simulink model "TrialAOOR"  (R2021a)
settings: Solver=FixedStepAuto  StartTime=0.0  StopTime=50  FixedStep=1e-3  RelTol=1e-3  EnableMultiTasking=on
undefined symbols (not defined in the file): D0, D1, D10, D11, D12, D13, D2, D3, D4, D5, D6, D7, D8, D9, magnitude, PTA0, PTA1, PTA2, PTB23, PTB9, PTC16, PTC17, PTC2, PTC3, PTC4, PTD0, PTD1, PTD2, PTD3
libraries: frdmk64flib x19, dspstat3 x1
settings Model: PacingRate=0.250000  ExtModeTrigDuration=5  Creator=Arun Mistry  LastModifiedBy=Arun Mistry
settings OptimizationCC: EnhancedBackFolding=on  PassReuseOutputArgsAs=Individual arguments  ZeroExternalMemoryAtStartup=off  ZeroInternalMemoryAtStartup=off  MaxStackSize=64  OptimizeBlockOrder=speed  DifferentSizesBufferReuse=on  OptimizationCustomize=off  EfficientTunableParamExpr=on
settings DebuggingCC: ParameterTunabilityLossMsg=error
settings HardwareCC: ProdBitPerPointer=32  ProdBitPerSizeT=32  ProdBitPerPtrDiffT=32  ProdLargestAtomicInteger=Long  ProdLargestAtomicFloat=Double  ProdWordSize=32  ProdHWDeviceType=ARM Compatible->ARM Cortex
settings SFSimCC: MATLABDynamicMemAlloc=off
settings RTWCC: SystemTargetFile=ert.tlc  HardwareBoard=NXP FRDM-K64F  TLCOptions="-aInlineSetEventsForThisBaseRateFcn=TLC_FALSE -aSuppressMultiTaskScheduler=TLC_FALSE  -aRateBasedStepFcn=0"  TemplateMakefile=ert_default_tmf  Toolchain=GNU Tools for ARM Embedded Processors
settings CodeAppCC: ForceParamTrailComments=on  IgnoreCustomStorageClasses=off  OperatorAnnotations=on  SimulinkDataObjDesc=on  SFDataObjDesc=on  InsertBlockDesc=on
settings ERTTargetCC: ExtModeTransport=4  ExtModeMexFile=sendToCommService

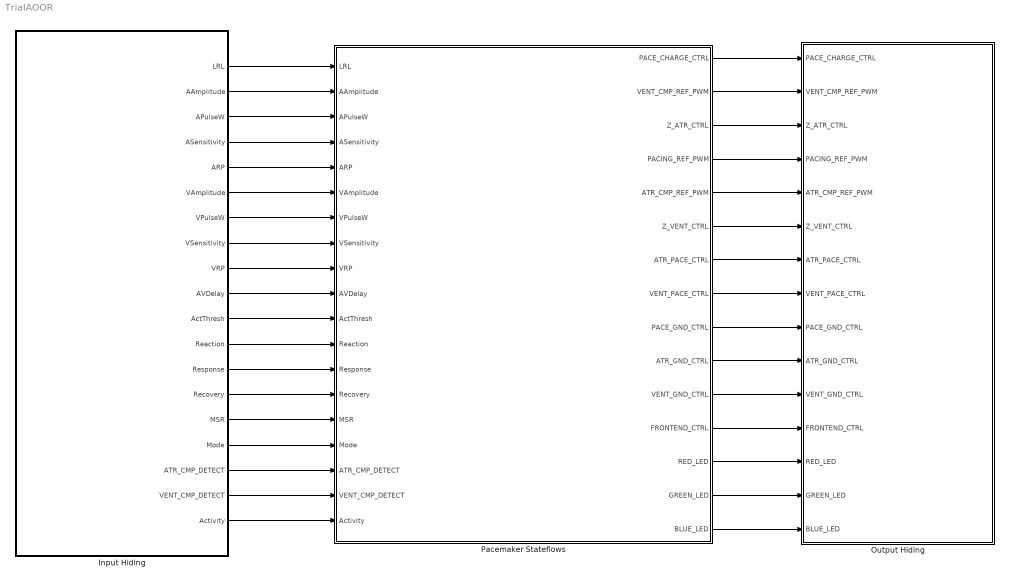
== system TrialAOOR ==
  Input Hiding : Subsystem
  Output Hiding : Subsystem
  Pacemaker Stateflows : Stateflow chart  TreatAsAtomicUnit=on
      settings: PortSchema="{\"entries\":[{\"content\":{\"sides\":[{\"content\":{\"connectorIds\":[\"In1\",\"In2\",\"In3\",\"In4\",\"In5\",\"In6\",\"In7\",\"In8\",\"In9\",\"In17\",\"In11\",\"In10\",\"In12\",\"In14\",\"In19\",\"In13\",\"In15\",\"In16\",\"In18\"]},\"type\":\"ConnectorPlacement.EquallySpacedRectSide\",\"uuid\":\"6f24296b-9994-4871-8227-e053a3629335\"},{\"content\":{\"connectorIds\":[\"Out1\",\"Out2\",\"Out3\",\"Out4\",\"Out5\",\"Out6\",\"Out7\",\"Out8\",\"Out9\",\"Out10\",\"Out11\",\"Out12\",\"Out13\",\"Out14\",\"Out15\"],\"side\":\"RIGHT\"},\"type\":\"ConnectorPlacement.EquallySpacedRectSide\",\"uuid\":\"36cf1f29-c3ea-48aa-b003-da737efff16a\"},{\"content\":{\"connectorIds\":[],\"side\":\"TOP\"},\"type\":\"ConnectorPlacement.EquallySpacedRectSide\",\"uuid\":\"8330eb51-0bc3-4d96-96ed-331fbb159cdb\"}]},\"type\":\"ConnectorPlacement.EquallySpacedConnector\",\"uuid\":\"1e79ed8a-065e-4a3c-97dd-23eb49490e0b\"}],\"packageUris\":[\"http://schema.mathworks.com/mf0/Connector/R2020b\"],\"version\":\"1.0\"}"
  wires:
  Pacemaker Stateflows/1(PACE_CHARGE_CTRL) -> Output Hiding/1(PACE_CHARGE_CTRL)
  Input Hiding/17(ATR_CMP_DETECT) -> Pacemaker Stateflows/15(ATR_CMP_DETECT)
  Input Hiding/7(VPulseW) -> Pacemaker Stateflows/7(VPulseW)
  Input Hiding/18(VENT_CMP_DETECT) -> Pacemaker Stateflows/16(VENT_CMP_DETECT)
  Pacemaker Stateflows/3(Z_ATR_CTRL) -> Output Hiding/3(Z_ATR_CTRL)
  Input Hiding/3(APulseW) -> Pacemaker Stateflows/3(APulseW)
  Pacemaker Stateflows/7(ATR_PACE_CTRL) -> Output Hiding/7(ATR_PACE_CTRL)
  Pacemaker Stateflows/10(ATR_GND_CTRL) -> Output Hiding/10(ATR_GND_CTRL)
  Input Hiding/16(Mode) -> Pacemaker Stateflows/13(Mode)
  Input Hiding/2(AAmplitude) -> Pacemaker Stateflows/2(AAmplitude)
  Input Hiding/6(VAmplitude) -> Pacemaker Stateflows/6(VAmplitude)
  Pacemaker Stateflows/6(Z_VENT_CTRL) -> Output Hiding/6(Z_VENT_CTRL)
  Pacemaker Stateflows/4(PACING_REF_PWM) -> Output Hiding/4(PACING_REF_PWM)
  Pacemaker Stateflows/11(VENT_GND_CTRL) -> Output Hiding/11(VENT_GND_CTRL)
  Pacemaker Stateflows/9(PACE_GND_CTRL) -> Output Hiding/9(PACE_GND_CTRL)
  Pacemaker Stateflows/8(VENT_PACE_CTRL) -> Output Hiding/8(VENT_PACE_CTRL)
  Input Hiding/1(LRL) -> Pacemaker Stateflows/1(LRL)
  Pacemaker Stateflows/15(BLUE_LED) -> Output Hiding/15(BLUE_LED)
  Input Hiding/4(ASensitivity) -> Pacemaker Stateflows/4(ASensitivity)
  Pacemaker Stateflows/12(FRONTEND_CTRL) -> Output Hiding/12(FRONTEND_CTRL)
  Input Hiding/9(VRP) -> Pacemaker Stateflows/9(VRP)
  Input Hiding/8(VSensitivity) -> Pacemaker Stateflows/8(VSensitivity)
  Input Hiding/5(ARP) -> Pacemaker Stateflows/5(ARP)
  Pacemaker Stateflows/14(GREEN_LED) -> Output Hiding/14(GREEN_LED)
  Pacemaker Stateflows/13(RED_LED) -> Output Hiding/13(RED_LED)
  Pacemaker Stateflows/5(ATR_CMP_REF_PWM) -> Output Hiding/5(ATR_CMP_REF_PWM)
  Pacemaker Stateflows/2(VENT_CMP_REF_PWM) -> Output Hiding/2(VENT_CMP_REF_PWM)
  Input Hiding/10(AVDelay) -> Pacemaker Stateflows/17(AVDelay)
  Input Hiding/19(Activity) -> Pacemaker Stateflows/18(Activity)
  Input Hiding/12(Reaction) -> Pacemaker Stateflows/10(Reaction)
  Input Hiding/13(Response) -> Pacemaker Stateflows/12(Response)
  Input Hiding/14(Recovery) -> Pacemaker Stateflows/14(Recovery)
  Input Hiding/15(MSR) -> Pacemaker Stateflows/19(MSR)
  Input Hiding/11(ActThresh) -> Pacemaker Stateflows/11(ActThresh)

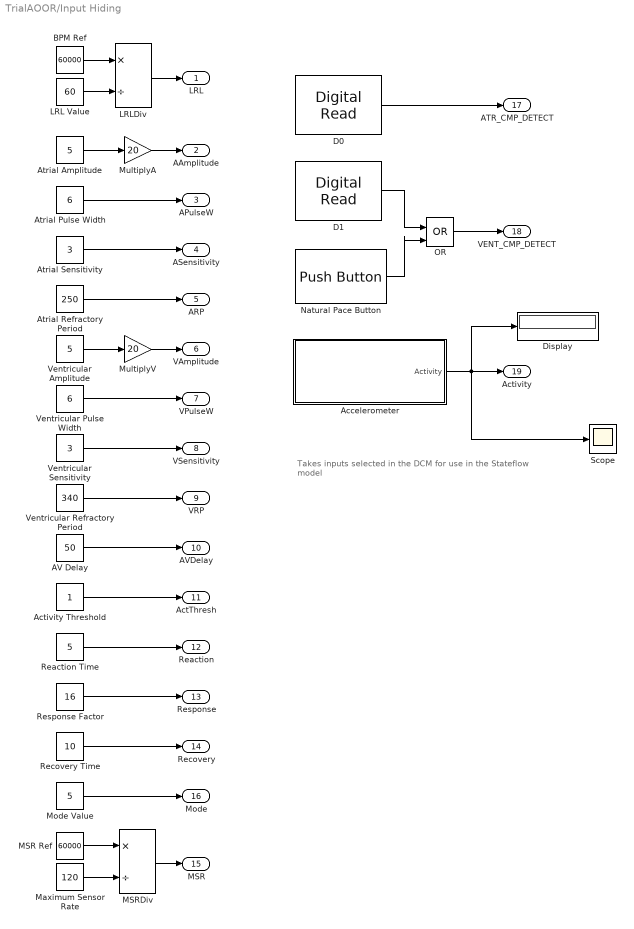
== system TrialAOOR/Input Hiding ==
  note: Takes inputs selected in the DCM for use in the Stateflow model
  AV Delay : Constant  Value=50  OutDataTypeStr=uint16
  Accelerometer : Subsystem
  Activity Threshold : Constant  OutDataTypeStr=double
  Atrial Amplitude : Constant  Value=5  OutDataTypeStr=uint16
  Atrial Pulse Width : Constant  Value=6  OutDataTypeStr=uint16
  Atrial Refractory Period : Constant  Value=250  OutDataTypeStr=uint16
  Atrial Sensitivity : Constant  Value=3  OutDataTypeStr=uint16
  BPM Ref : Constant  Value=60000  OutDataTypeStr=uint16
  D0 : frdmk64flib/Digital Read  Whichpin=PTC16 (D0)  SampleTime=-1
  D1 : frdmk64flib/Digital Read  Whichpin=PTC17 (D1)  SampleTime=-1
  Display : Display
  LRL Value : Constant  Value=60  OutDataTypeStr=uint16
  LRLDiv : Product  Inputs=*/  OutDataTypeStr=uint16  RndMeth=Round
  MSR Ref : Constant  Value=60000  OutDataTypeStr=uint16
  MSRDiv : Product  Inputs=*/  OutDataTypeStr=uint16  RndMeth=Round
  Maximum Sensor Rate : Constant  Value=120  OutDataTypeStr=uint16
  Mode Value : Constant  Value=5  OutDataTypeStr=uint16
  MultiplyA : Gain  Gain=20  OutDataTypeStr=uint16
  MultiplyV : Gain  Gain=20  OutDataTypeStr=uint16
  Natural Pace Button : frdmk64flib/Push Button  Whichswitch=SW3  SampleTime1=-1
  OR : Logic  Operator=OR  IconShape=distinctive  AllPortsSameDT=off  OutDataTypeStr=boolean
  Reaction Time : Constant  Value=5  OutDataTypeStr=uint16
  Recovery Time : Constant  Value=10  OutDataTypeStr=uint16
  Response Factor : Constant  Value=16  OutDataTypeStr=uint16
  Scope : Scope
  Ventricular Amplitude : Constant  Value=5  OutDataTypeStr=uint16
  Ventricular Pulse Width : Constant  Value=6  OutDataTypeStr=uint16
  Ventricular Refractory Period : Constant  Value=340  OutDataTypeStr=uint16
  Ventricular Sensitivity : Constant  Value=3  OutDataTypeStr=uint16
  LRL : Outport  OutDataTypeStr=uint16
  AAmplitude : Outport  Port=2  OutDataTypeStr=uint16
  APulseW : Outport  Port=3  OutDataTypeStr=uint16
  ASensitivity : Outport  Port=4  OutDataTypeStr=uint16
  ARP : Outport  Port=5  OutDataTypeStr=uint16
  VAmplitude : Outport  Port=6  OutDataTypeStr=uint16
  VPulseW : Outport  Port=7  OutDataTypeStr=uint16
  VSensitivity : Outport  Port=8  OutDataTypeStr=uint16
  VRP : Outport  Port=9  OutDataTypeStr=uint16
  AVDelay : Outport  Port=10  OutDataTypeStr=uint16
  ActThresh : Outport  Port=11  OutDataTypeStr=double
  Reaction : Outport  Port=12  OutDataTypeStr=uint16
  Response : Outport  Port=13  OutDataTypeStr=uint16
  Recovery : Outport  Port=14  OutDataTypeStr=uint16
  MSR : Outport  Port=15  OutDataTypeStr=uint16
  Mode : Outport  Port=16  OutDataTypeStr=uint16
  ATR_CMP_DETECT : Outport  Port=17  OutDataTypeStr=boolean
  VENT_CMP_DETECT : Outport  Port=18  OutDataTypeStr=boolean
  Activity : Outport  Port=19
  wires:
  Atrial Amplitude/1 -> MultiplyA/1
  Ventricular Amplitude/1 -> MultiplyV/1
  Atrial Pulse Width/1 -> APulseW/1
  Ventricular Pulse Width/1 -> VPulseW/1
  Atrial Sensitivity/1 -> ASensitivity/1
  Ventricular Sensitivity/1 -> VSensitivity/1
  Ventricular Refractory Period/1 -> VRP/1
  Atrial Refractory Period/1 -> ARP/1
  D0/1 -> ATR_CMP_DETECT/1
  Natural Pace Button/1 -> OR/2
  Mode Value/1 -> Mode/1
  BPM Ref/1 -> LRLDiv/1
  LRLDiv/1 -> LRL/1
  D1/1 -> OR/1
  OR/1 -> VENT_CMP_DETECT/1
  AV Delay/1 -> AVDelay/1
  LRL Value/1 -> LRLDiv/2
  MultiplyV/1 -> VAmplitude/1
  MultiplyA/1 -> AAmplitude/1
  Accelerometer/1(Activity) -> Display/1, Activity/1, Scope/1
  Reaction Time/1 -> Reaction/1
  Response Factor/1 -> Response/1
  Recovery Time/1 -> Recovery/1
  Maximum Sensor Rate/1 -> MSRDiv/2
  MSR Ref/1 -> MSRDiv/1
  MSRDiv/1 -> MSR/1
  Activity Threshold/1 -> ActThresh/1

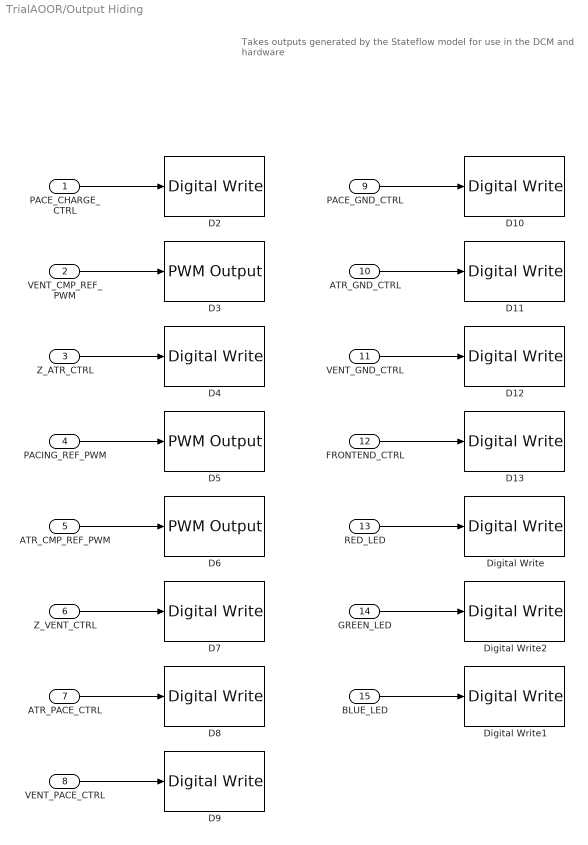
== system TrialAOOR/Output Hiding ==
  note: Takes outputs generated by the Stateflow model for use in the DCM and hardware
  PACE_CHARGE_CTRL : Inport  OutDataTypeStr=uint16
  VENT_CMP_REF_PWM : Inport  Port=2  OutDataTypeStr=uint16
  Z_ATR_CTRL : Inport  Port=3  OutDataTypeStr=uint16
  PACING_REF_PWM : Inport  Port=4  OutDataTypeStr=uint16
  ATR_CMP_REF_PWM : Inport  Port=5  OutDataTypeStr=uint16
  Z_VENT_CTRL : Inport  Port=6  OutDataTypeStr=uint16
  ATR_PACE_CTRL : Inport  Port=7  OutDataTypeStr=uint16
  VENT_PACE_CTRL : Inport  Port=8  OutDataTypeStr=uint16
  PACE_GND_CTRL : Inport  Port=9  OutDataTypeStr=uint16
  ATR_GND_CTRL : Inport  Port=10  OutDataTypeStr=uint16
  VENT_GND_CTRL : Inport  Port=11  OutDataTypeStr=uint16
  FRONTEND_CTRL : Inport  Port=12  OutDataTypeStr=uint16
  RED_LED : Inport  Port=13  OutDataTypeStr=uint16
  GREEN_LED : Inport  Port=14  OutDataTypeStr=uint16
  BLUE_LED : Inport  Port=15  OutDataTypeStr=uint16
  D10 : frdmk64flib/Digital Write  Whichpin=PTD0 (D10)
  D11 : frdmk64flib/Digital Write  Whichpin=PTD2 (D11)
  D12 : frdmk64flib/Digital Write  Whichpin=PTD3 (D12)
  D13 : frdmk64flib/Digital Write  Whichpin=PTD1 (D13)
  D2 : frdmk64flib/Digital Write  Whichpin=PTB9 (D2)
  D3 : frdmk64flib/PWM Output  Whichpin=PTA1 (D3)  InitialFrequency=2000  InitialDutyCycle=100
  D4 : frdmk64flib/Digital Write  Whichpin=PTB23 (D4)
  D5 : frdmk64flib/PWM Output  Whichpin=PTA2 (D5)  InitialFrequency=2000  InitialDutyCycle=100
  D6 : frdmk64flib/PWM Output  Whichpin=PTC2 (D6)  InitialFrequency=2000  InitialDutyCycle=100
  D7 : frdmk64flib/Digital Write  Whichpin=PTC3 (D7)
  "D8 " : frdmk64flib/Digital Write  Whichpin=PTA0 (D8)
  D9 : frdmk64flib/Digital Write  Whichpin=PTC4 (D9)
  Digital Write : frdmk64flib/Digital Write  Whichpin=RED_LED
  Digital Write1 : frdmk64flib/Digital Write  Whichpin=BLUE_LED
  Digital Write2 : frdmk64flib/Digital Write  Whichpin=GREEN_LED
  wires:
  VENT_PACE_CTRL/1 -> D9/1
  ATR_CMP_REF_PWM/1 -> D6/1
  PACE_GND_CTRL/1 -> D10/1
  VENT_CMP_REF_PWM/1 -> D3/1
  PACING_REF_PWM/1 -> D5/1
  ATR_GND_CTRL/1 -> D11/1
  ATR_PACE_CTRL/1 -> "D8 "/1
  PACE_CHARGE_CTRL/1 -> D2/1
  FRONTEND_CTRL/1 -> D13/1
  VENT_GND_CTRL/1 -> D12/1
  Z_ATR_CTRL/1 -> D4/1
  Z_VENT_CTRL/1 -> D7/1
  RED_LED/1 -> Digital Write/1
  BLUE_LED/1 -> Digital Write1/1
  GREEN_LED/1 -> Digital Write2/1

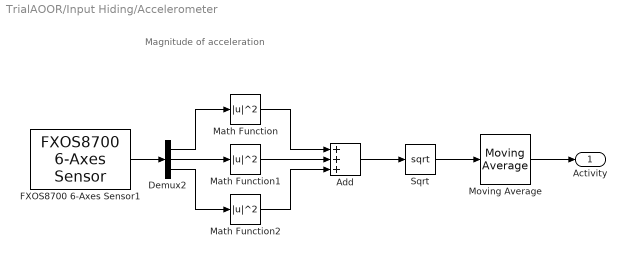
== system TrialAOOR/Input Hiding/Accelerometer ==
  note: Magnitude of acceleration
  Add : Sum  Inputs=+++
  Demux2 : Demux  Outputs=3
  FXOS8700 6-Axes Sensor1 : frdmk64flib/FXOS8700 6-Axes Sensor  Activesensor=Accelerometer only  ODR=100Hz  HybridODR=400Hz  Accelfullrange=-4g to +4g  SampleTime=1/100
  Math Function : Math  Operator=magnitude^2  SignedPower=on  OutDataTypeStr=double  SaturateOnIntegerOverflow=on
  Math Function1 : Math  Operator=magnitude^2  SignedPower=on  OutDataTypeStr=double  SaturateOnIntegerOverflow=on
  Math Function2 : Math  Operator=magnitude^2  SignedPower=on  OutDataTypeStr=double  SaturateOnIntegerOverflow=on
  Moving Average : dspstat3/Moving Average  Method=Sliding window  ForgettingFactorPort=off  SpecifyWindowLength=on  WindowLength=30  ForgettingFactor=0.9  SimulateUsing=Code generation
  Sqrt : Sqrt  SaturateOnIntegerOverflow=on
  Activity : Outport  OutDataTypeStr=double  SourceOfInitialOutputValue=Input signal
  wires:
  Sqrt/1 -> Moving Average/1
  FXOS8700 6-Axes Sensor1/1 -> Demux2/1
  Math Function/1 -> Add/1
  Add/1 -> Sqrt/1
  Math Function2/1 -> Add/3
  Demux2/2 -> Math Function1/1
  Math Function1/1 -> Add/2
  Demux2/1 -> Math Function/1
  Demux2/3 -> Math Function2/1
  Moving Average/1 -> Activity/1

== stateflow chart TrialAOOR/Pacemaker Stateflows ==
  note: Mode selected from DCM changes which State will be run
  state AOO [commented out]
    entry:
    VENT_PACE_CTRL = 0; VENT_GND_CTRL = 0; PACE_GND_CTRL = 1;
    Z_VENT_CTRL = 0; Z_ATR_CTRL = 0; PACING_REF_PWM = AAmplitude;
    note: Duration of Pulse
    state PACE_ATR [commented out]
      entry:
      PACE_CHARGE_CTRL = 0;
      ATR_GND_CTRL = 0;
      ATR_PACE_CTRL = 1;
      RED_LED = 1;
    state C22_CHARGE [commented out]
      entry:
      PACE_CHARGE_CTRL = 1;
      ATR_PACE_CTRL = 0;
      ATR_GND_CTRL = 1;
      RED_LED = 0;
    note: Wait for LRL before Pulse
    note: Toggle values between
        | C22_CHARGE and PACE_ATR
    (default) -> AOO.C22_CHARGE [commented out]
    AOO.PACE_ATR -> AOO.C22_CHARGE [commented out] : after(APulseW,msec)
    AOO.C22_CHARGE -> AOO.PACE_ATR [commented out] : after(LRL-APulseW,msec)
  state MODE_SELECTION
    entry:
    GREEN_LED = 0;
    RED_LED = 0;
    BLUE_LED = 0;
    FRONTEND_CTRL = 0;
    PACING_REF_PWM = 0;
    ATR_CMP_REF_PWM = 0;
    VENT_CMP_REF_PWM = 0;
    PACE_CHARGE_CTRL= 0;
    PACE_GND_CTRL= 0;
    ATR_PACE_CTRL = 0;
    ATR_GND_CTRL = 0;
    VENT_PACE_CTRL = 0;
    VENT_GND_CTRL = 0;
    Z_ATR_CTRL = 0;
    Z_VENT_CTRL = 0;
    note: Reset the values above
        | upon switching modes
  state VOO [commented out]
    entry:
    ATR_PACE_CTRL = 0; ATR_GND_CTRL = 0; PACE_GND_CTRL = 1;
    Z_ATR_CTRL = 0; Z_VENT_CTRL = 0; PACING_REF_PWM = VAmplitude;
    note: Duration of high
    state PACE_VENT [commented out]
      entry:
      PACE_CHARGE_CTRL = 0;
      VENT_GND_CTRL = 0;
      VENT_PACE_CTRL = 1;
      BLUE_LED = 1;
    state C22_CHARGE [commented out]
      entry:
      VENT_PACE_CTRL = 0;
      VENT_GND_CTRL = 1;
      PACE_CHARGE_CTRL = 1;
      BLUE_LED = 0;
    note: Duration of low
    note: Toggle values between
        | C22_CHARGE and PACE_VENT
    (default) -> VOO.C22_CHARGE [commented out]
    VOO.PACE_VENT -> VOO.C22_CHARGE [commented out] : after(VPulseW,msec)
    VOO.C22_CHARGE -> VOO.PACE_VENT [commented out] : after(LRL-VPulseW,msec)
  note: Mode 1
  note: Mode 2
  state AAI [commented out]
    entry:
    VENT_PACE_CTRL = 0; VENT_GND_CTRL = 0; ATR_CMP_REF_PWM = ASensitivity;
    Z_VENT_CTRL = 0; Z_ATR_CTRL = 0;PACING_REF_PWM = AAmplitude;PACE_GND_CTRL = 1;FRONTEND_CTRL = 1; sense = 0;
    state C22_CHARGE [commented out]
      entry:
      RED_LED = 0;
      PACE_CHARGE_CTRL = 1;
      ATR_GND_CTRL = 1;
      ATR_PACE_CTRL = 0;
      sense = 0;
    state PACE_ATR [commented out]
      entry:
      RED_LED = 1;
      PACE_CHARGE_CTRL = 0;
      ATR_GND_CTRL = 0;
      ATR_PACE_CTRL = 1;
      sense = 1;
    state REFRACTORY [commented out]
      entry:
      GREEN_LED = 1;
      PACE_CHARGE_CTRL = 1;
      ATR_GND_CTRL = 1;
      ATR_PACE_CTRL = 0;
    (default) -> AAI.C22_CHARGE [commented out]
    AAI.REFRACTORY -> AAI.C22_CHARGE [commented out] : after(ARP-(APulseW * sense),msec)
    AAI.C22_CHARGE -> AAI.PACE_ATR [commented out] : after(LRL-ARP,msec)
    AAI.PACE_ATR -> AAI.REFRACTORY [commented out] : after(APulseW,msec)
    AAI.C22_CHARGE -> AAI.REFRACTORY [commented out] : [ATR_CMP_DETECT == true]
  state VVI [commented out]
    entry:
    ATR_PACE_CTRL = 0; ATR_GND_CTRL = 0; PACE_GND_CTRL = 1; VENT_CMP_REF_PWM = VSensitivity;
    Z_VENT_CTRL = 0; Z_ATR_CTRL = 0;FRONTEND_CTRL = 1; PACING_REF_PWM = VAmplitude; sense = 0;
    state PACE_VENT [commented out]
      entry:
      BLUE_LED = 1;
      PACE_CHARGE_CTRL = 0;
      VENT_GND_CTRL = 0;
      VENT_PACE_CTRL = 1;
      sense = 1;
    state C22_CHARGE [commented out]
      entry:
      BLUE_LED = 0;
      PACE_CHARGE_CTRL = 1;
      VENT_GND_CTRL = 1;
      VENT_PACE_CTRL = 0;
      sense = 0;
    state REFRACTORY [commented out]
      entry:
      GREEN_LED = 1;
      PACE_CHARGE_CTRL = 1;
      VENT_GND_CTRL = 1;
      VENT_PACE_CTRL = 0;
    (default) -> VVI.C22_CHARGE [commented out]
    VVI.C22_CHARGE -> VVI.PACE_VENT [commented out] : after(LRL-VRP,msec)
    VVI.REFRACTORY -> VVI.C22_CHARGE [commented out] : after(VRP-(VPulseW *sense),msec)
    VVI.PACE_VENT -> VVI.REFRACTORY [commented out] : after(VPulseW,msec)
    VVI.C22_CHARGE -> VVI.REFRACTORY [commented out] : [VENT_CMP_DETECT == true]
  note: Mode 3
  note: Mode 4
  state AOOR
    entry:
    Z_VENT_CTRL = 0;
    Z_ATR_CTRL = 0;
    VENT_PACE_CTRL = 0;
    VENT_GND_CTRL = 0;
    PACE_GND_CTRL = 1;
    PACING_REF_PWM = AAmplitude;
    state PACE [parallel]
      settings: executionOrder=1
      state PACE_ATR
        entry:
        PACE_CHARGE_CTRL = 0;
        ATR_GND_CTRL = 0;
        ATR_PACE_CTRL = 1;
        RED_LED = 1;
      state C22_CHARGE
        entry:
        PACE_CHARGE_CTRL = 1;
        ATR_PACE_CTRL = 0;
        ATR_GND_CTRL = 1;
        RED_LED = 0;
      (default) -> AOOR.PACE.C22_CHARGE
      AOOR.PACE.PACE_ATR -> AOOR.PACE.C22_CHARGE : after(APulseW,msec)
      AOOR.PACE.C22_CHARGE -> AOOR.PACE.PACE_ATR : after(ModRate-APulseW,msec)
    state MODULATION [parallel]
      entry: increment = (LRL-MSR)/Reaction; decrement = (LRL-MSR)/Recovery;
      during: Target = LRL - (Activity - ActThresh)/(17 - Response*0.9)*2500;
      settings: executionOrder=2
      state STEPUP
        entry:
        ModRate = ModRate - increment/100;
      state START
        entry:
        ModRate = LRL;
      state MAXIMUM
        entry:
        ModRate = MSR;
      state STEPDOWN
        entry:
        ModRate = ModRate + decrement/100;
      STEPUP -> STEPUP [order 2] : after(10,msec)[ModRate > Target]
      START -> STEPUP : [Target < LRL]
      STEPUP -> MAXIMUM [order 1] : [ModRate <= MSR]
      STEPUP -> STEPDOWN [order 3] : after(10,msec)
          | [ModRate <= Target]
      STEPDOWN -> STEPUP [order 3] : after(10,msec)
          | [ModRate >= Target]
      (default) -> START
      STEPDOWN -> START [order 1] : [ModRate >= LRL]
      MAXIMUM -> STEPDOWN : [Target > MSR]
      STEPDOWN -> STEPDOWN [order 2] : after(10, msec)[ModRate < Target]
  state VOOR [commented out]
    entry:
    ATR_PACE_CTRL = 0; ATR_GND_CTRL = 0; PACE_GND_CTRL = 1;
    Z_ATR_CTRL = 0; Z_VENT_CTRL = 0; PACING_REF_PWM = VAmplitude;
    during: ModRate = Modulation(LRL,MSR,Activity,Reaction,Response,Recovery);
    state PACE_VENT [commented out]
      entry:
      PACE_CHARGE_CTRL = 0;
      VENT_GND_CTRL = 0;
      VENT_PACE_CTRL = 1;
      BLUE_LED = 1;
    state C22_CHARGE [commented out]
      entry:
      VENT_PACE_CTRL = 0;
      VENT_GND_CTRL = 1;
      PACE_CHARGE_CTRL = 1;
      BLUE_LED = 0;
    (default) -> VOOR.C22_CHARGE [commented out]
    VOOR.PACE_VENT -> VOOR.C22_CHARGE [commented out] : after(VPulseW,msec)
    VOOR.C22_CHARGE -> VOOR.PACE_VENT [commented out] : after(ModRate-VPulseW,msec)
  note: Mode 5
  note: Mode 6
  state AAIR [commented out]
    entry:
    VENT_PACE_CTRL = 0; VENT_GND_CTRL = 0; ATR_CMP_REF_PWM = 70;
    Z_VENT_CTRL = 0; Z_ATR_CTRL = 0;PACING_REF_PWM = AAmplitude;PACE_GND_CTRL = 1;FRONTEND_CTRL = 1; sense = 0;
    state C22_CHARGE [commented out]
      entry:
      RED_LED = 0;
      PACE_CHARGE_CTRL = 1;
      ATR_GND_CTRL = 1;
      ATR_PACE_CTRL = 0;
      sense = 0;
    state PACE_ATR [commented out]
      entry:
      RED_LED = 1;
      PACE_CHARGE_CTRL = 0;
      ATR_GND_CTRL = 0;
      ATR_PACE_CTRL = 1;
      sense = 1;
    state REFRACTORY [commented out]
      entry:
      GREEN_LED = 1;
      PACE_CHARGE_CTRL = 1;
      ATR_GND_CTRL = 1;
      ATR_PACE_CTRL = 0;
    (default) -> AAIR.C22_CHARGE [commented out]
    AAIR.REFRACTORY -> AAIR.C22_CHARGE [commented out] : after(ARP-(APulseW * sense),msec)
    AAIR.C22_CHARGE -> AAIR.PACE_ATR [commented out] : after(ModRate-ARP,msec)
    AAIR.PACE_ATR -> AAIR.REFRACTORY [commented out] : after(APulseW,msec)
    AAIR.C22_CHARGE -> AAIR.REFRACTORY [commented out] : [ATR_CMP_DETECT == true]
  state VVIR [commented out]
    entry:
    ATR_PACE_CTRL = 0; ATR_GND_CTRL = 0; PACE_GND_CTRL = 1; VENT_CMP_REF_PWM = 70;
    Z_VENT_CTRL = 0; Z_ATR_CTRL = 0;FRONTEND_CTRL = 1; PACING_REF_PWM = VAmplitude; sense = 0;
    state PACE_VENT [commented out]
      entry:
      BLUE_LED = 1;
      PACE_CHARGE_CTRL = 0;
      VENT_GND_CTRL = 0;
      VENT_PACE_CTRL = 1;
      sense = 1;
    state C22_CHARGE [commented out]
      entry:
      BLUE_LED = 0;
      PACE_CHARGE_CTRL = 1;
      VENT_GND_CTRL = 1;
      VENT_PACE_CTRL = 0;
      sense = 0;
    state REFRACTORY [commented out]
      entry:
      GREEN_LED = 1;
      PACE_CHARGE_CTRL = 1;
      VENT_GND_CTRL = 1;
      VENT_PACE_CTRL = 0;
    (default) -> VVIR.C22_CHARGE [commented out]
    VVIR.C22_CHARGE -> VVIR.PACE_VENT [commented out] : after(ModRate-VRP,msec)
    VVIR.REFRACTORY -> VVIR.C22_CHARGE [commented out] : after(VRP-(VPulseW *sense),msec)
    VVIR.PACE_VENT -> VVIR.REFRACTORY [commented out] : after(VPulseW,msec)
    VVIR.C22_CHARGE -> VVIR.REFRACTORY [commented out] : [VENT_CMP_DETECT == true]
  note: Mode 7
  note: Mode 8
  state DOO [commented out]
    entry:
    Z_VENT_CTRL = 0; Z_ATR_CTRL = 0; PACE_GND_CTRL = 1;
    note: Both low,
        | prep for ATR pulse
    note: Pace ATR
    state PACE_ATR [commented out]
      entry:
      PACE_CHARGE_CTRL = 0;
      ATR_GND_CTRL = 0;
      VENT_GND_CTRL = 0;
      ATR_PACE_CTRL = 1;
      RED_LED = 1;
    state C22_CHARGE [commented out]
      entry:
      ATR_PACE_CTRL = 0;
      VENT_PACE_CTRL = 0;
      PACING_REF_PWM = AAmplitude;
      PACE_CHARGE_CTRL = 1;
      ATR_GND_CTRL = 0;
      VENT_GND_CTRL = 1;
      BLUE_LED = 0;
    note: Duration of ATR pulse high
    note: Duration of VENT pulse high
    state AVDelay_PERIOD [commented out]
      entry:
      ATR_PACE_CTRL = 0;
      VENT_PACE_CTRL = 0;
      PACING_REF_PWM = VAmplitude;
      PACE_CHARGE_CTRL = 1;
      ATR_GND_CTRL = 1;
      VENT_GND_CTRL = 0;
      RED_LED = 0;
    state PACE_VENT [commented out]
      entry:
      PACE_CHARGE_CTRL = 0;
      ATR_GND_CTRL = 0;
      VENT_GND_CTRL = 0;
      VENT_PACE_CTRL = 1;
      BLUE_LED = 1;
    note: Pace vent
    note: Both low,
        | prep for VENT pulse
    (default) -> DOO.C22_CHARGE [commented out]
    DOO.C22_CHARGE -> DOO.PACE_ATR [commented out] : after(LRL-AVDelay-VPulseW,msec)
    DOO.PACE_ATR -> DOO.AVDelay_PERIOD [commented out] : after(APulseW,msec)
    DOO.PACE_VENT -> DOO.C22_CHARGE [commented out] : after(VPulseW, msec)
    DOO.AVDelay_PERIOD -> DOO.PACE_VENT [commented out] : after(AVDelay-APulseW,msec)
  state DOOR [commented out]
    entry:
    Z_VENT_CTRL = 0; Z_ATR_CTRL = 0; PACE_GND_CTRL = 1;
    state C22_CHARGE [commented out]
      entry:
      ATR_PACE_CTRL = 0;
      VENT_PACE_CTRL = 0;
      PACING_REF_PWM = AAmplitude*20;
      PACE_CHARGE_CTRL = 1;
      ATR_GND_CTRL = 0;
      VENT_GND_CTRL = 1;
      BLUE_LED = 0;
    state PACE_ATR [commented out]
      entry:
      PACE_CHARGE_CTRL = 0;
      ATR_GND_CTRL = 0;
      VENT_GND_CTRL = 0;
      ATR_PACE_CTRL = 1;
      RED_LED = 1;
    state AVDelay_PERIOD [commented out]
      entry:
      ATR_PACE_CTRL = 0;
      VENT_PACE_CTRL = 0;
      PACING_REF_PWM = VAmplitude*20;
      PACE_CHARGE_CTRL = 1;
      ATR_GND_CTRL = 1;
      VENT_GND_CTRL = 0;
      RED_LED = 0;
      BLUE_LED = 0;
    state PACE_VENT [commented out]
      entry:
      PACE_CHARGE_CTRL = 0;
      ATR_GND_CTRL = 0;
      VENT_GND_CTRL = 0;
      VENT_PACE_CTRL = 1;
      BLUE_LED = 1;
    (default) -> DOOR.C22_CHARGE [commented out]
    DOOR.C22_CHARGE -> DOOR.PACE_ATR [commented out] : after(ModRate-AVDelay-VPulseW,msec)
    DOOR.PACE_ATR -> DOOR.AVDelay_PERIOD [commented out] : after(APulseW,msec)
    DOOR.PACE_VENT -> DOOR.C22_CHARGE [commented out] : after(VPulseW, msec)
    DOOR.AVDelay_PERIOD -> DOOR.PACE_VENT [commented out] : after(AVDelay-APulseW,msec)
  state DDD [commented out]
    entry:
    Z_VENT_CTRL = 0; Z_ATR_CTRL = 0; PACE_GND_CTRL = 1;
    state C22_CHARGE [commented out]
      entry:
      ATR_PACE_CTRL = 0;
      VENT_PACE_CTRL = 0;
      PACING_REF_PWM = AAmplitude*20;
      PACE_CHARGE_CTRL = 1;
      ATR_GND_CTRL = 0;
      VENT_GND_CTRL = 1;
      BLUE_LED = 0;
    state PACE_ATR [commented out]
      entry:
      PACE_CHARGE_CTRL = 0;
      ATR_GND_CTRL = 0;
      VENT_GND_CTRL = 0;
      ATR_PACE_CTRL = 1;
      RED_LED = 1;
    state AVDelay_PERIOD [commented out]
      entry:
      ATR_PACE_CTRL = 0;
      VENT_PACE_CTRL = 0;
      PACING_REF_PWM = VAmplitude*20;
      PACE_CHARGE_CTRL = 1;
      ATR_GND_CTRL = 1;
      VENT_GND_CTRL = 0;
      RED_LED = 0;
      BLUE_LED = 0;
    state PACE_VENT [commented out]
      entry:
      PACE_CHARGE_CTRL = 0;
      ATR_GND_CTRL = 0;
      VENT_GND_CTRL = 0;
      VENT_PACE_CTRL = 1;
      BLUE_LED = 1;
    (default) -> DDD.C22_CHARGE [commented out]
    DDD.C22_CHARGE -> DDD.PACE_ATR [commented out] : after(ModRate-AVDelay-VPulseW,msec)
    DDD.PACE_ATR -> DDD.AVDelay_PERIOD [commented out] : after(APulseW,msec)
    DDD.PACE_VENT -> DDD.C22_CHARGE [commented out] : after(VPulseW, msec)
    DDD.AVDelay_PERIOD -> DDD.PACE_VENT [commented out] : after(AVDelay-APulseW,msec)
  state DDDR [commented out]
    entry:
    Z_VENT_CTRL = 0; Z_ATR_CTRL = 0; PACE_GND_CTRL = 1;
    state C22_CHARGE [commented out]
      entry:
      ATR_PACE_CTRL = 0;
      VENT_PACE_CTRL = 0;
      PACING_REF_PWM = AAmplitude*20;
      PACE_CHARGE_CTRL = 1;
      ATR_GND_CTRL = 0;
      VENT_GND_CTRL = 1;
      BLUE_LED = 0;
    state PACE_ATR [commented out]
      entry:
      PACE_CHARGE_CTRL = 0;
      ATR_GND_CTRL = 0;
      VENT_GND_CTRL = 0;
      ATR_PACE_CTRL = 1;
      RED_LED = 1;
    state AVDelay_PERIOD [commented out]
      entry:
      ATR_PACE_CTRL = 0;
      VENT_PACE_CTRL = 0;
      PACING_REF_PWM = VAmplitude*20;
      PACE_CHARGE_CTRL = 1;
      ATR_GND_CTRL = 1;
      VENT_GND_CTRL = 0;
      RED_LED = 0;
      BLUE_LED = 0;
    state PACE_VENT [commented out]
      entry:
      PACE_CHARGE_CTRL = 0;
      ATR_GND_CTRL = 0;
      VENT_GND_CTRL = 0;
      VENT_PACE_CTRL = 1;
      BLUE_LED = 1;
    (default) -> DDDR.C22_CHARGE [commented out]
    DDDR.C22_CHARGE -> DDDR.PACE_ATR [commented out] : after(LRL-AVDelay-VPulseW,msec)
    DDDR.PACE_ATR -> DDDR.AVDelay_PERIOD [commented out] : after(APulseW,msec)
    DDDR.PACE_VENT -> DDDR.C22_CHARGE [commented out] : after(VPulseW, msec)
    DDDR.AVDelay_PERIOD -> DDDR.PACE_VENT [commented out] : after(AVDelay-APulseW,msec)
  note: Mode 9
  note: Mode 10
  note: Mode 11
  note: Mode 12
  (default) -> MODE_SELECTION
  MODE_SELECTION -> VOO [commented out] : [Mode==2]
  MODE_SELECTION -> AOO [commented out] : [Mode==1]
  VOO -> MODE_SELECTION [commented out] : [Mode~=2]
  AOO -> MODE_SELECTION [commented out] : [Mode~=1]
  MODE_SELECTION -> AAI [commented out] : [Mode==3]
  MODE_SELECTION -> VVI [commented out] : [Mode==4]
  AAI -> MODE_SELECTION [commented out] : [Mode~=3]
  VVI -> MODE_SELECTION [commented out] : [Mode~=4]
  MODE_SELECTION -> AOOR : [Mode==5]
  MODE_SELECTION -> VOOR [commented out] : [Mode==6]
  AOOR -> MODE_SELECTION : [Mode~=5]
  VOOR -> MODE_SELECTION [commented out] : [Mode~=6]
  MODE_SELECTION -> VVIR [commented out] : [Mode==8]
  MODE_SELECTION -> AAIR [commented out] : [Mode==7]
  AAIR -> MODE_SELECTION [commented out] : [Mode~=7]
  VVIR -> MODE_SELECTION [commented out] : [Mode~=8]
  MODE_SELECTION -> DOO [commented out] : [Mode==9]
  MODE_SELECTION -> DDDR [commented out] : [Mode==12]
  DOO -> MODE_SELECTION [commented out] : [Mode~=9]
  DDDR -> MODE_SELECTION [commented out] : [Mode~=12]
  MODE_SELECTION -> DOOR [commented out] : [Mode==10]
  DOOR -> MODE_SELECTION [commented out] : [Mode~=10]
  DDD -> MODE_SELECTION [commented out] : [Mode~=11]
  MODE_SELECTION -> DDD [commented out] : [Mode==11]
  data: LRL input uint16; AAmplitude input uint16; APulseW input uint16; ASensitivity input uint16; ARP input uint16; VAmplitude input uint16; VPulseW input uint16; VSensitivity input uint16; VRP input uint16; Reaction input; ActThresh input; Response input; PACE_CHARGE_CTRL output uint16; VENT_CMP_REF_PWM output uint16; Z_ATR_CTRL output uint16; PACING_REF_PWM output uint16; ATR_CMP_REF_PWM output uint16; Z_VENT_CTRL output uint16; ATR_PACE_CTRL output uint16; VENT_PACE_CTRL output uint16; PACE_GND_CTRL output uint16; ATR_GND_CTRL output uint16; VENT_GND_CTRL output uint16; Mode input uint16; Recovery input; FRONTEND_CTRL output uint16; RED_LED output uint16; GREEN_LED output uint16; BLUE_LED output uint16; ATR_CMP_DETECT input boolean; VENT_CMP_DETECT input boolean; AVDelay input uint16; sense local uint16; Activity input; ModRate local; MSR input; Target local; decrement local; increment local
